simulink model "notch"  (R2017a)
settings: Solver=VariableStepAuto  StartTime=0.0  StopTime=20  RelTol=1e-3
settings Model: Creator=Chaohua Zhao  LastModifiedBy=Chaohua Zhao

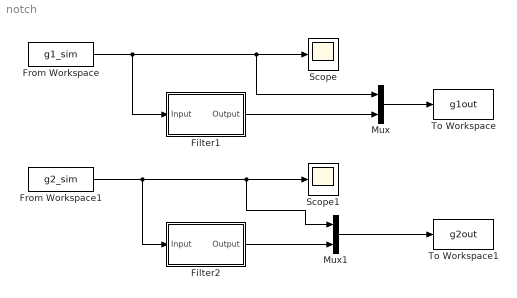
== system notch ==
  Filter1 : Subsystem  Tag=FilterWizardSubSystem
      settings: ErrorFcn=dspFilterRealizedInBasicElemsAlgLoopErrFcnCallback
  Filter2 : Subsystem  Tag=FilterWizardSubSystem
      settings: ErrorFcn=dspFilterRealizedInBasicElemsAlgLoopErrFcnCallback
  From Workspace : FromWorkspace  VariableName=g1_sim  SampleTime=0.001  OutputAfterFinalValue=Setting to zero
  From Workspace1 : FromWorkspace  VariableName=g2_sim  SampleTime=0.001  OutputAfterFinalValue=Setting to zero
  Mux : Mux  Inputs=2
  Mux1 : Mux  Inputs=2
  Scope : Scope
  Scope1 : Scope
  To Workspace : ToWorkspace  VariableName=g1out  SampleTime=-1
  To Workspace1 : ToWorkspace  VariableName=g2out  SampleTime=-1
  wires:
  From Workspace/1 -> Filter1/1(Input), Mux/1, Scope/1
  Filter1/1(Output) -> Mux/2
  Mux/1 -> To Workspace/1
  Filter2/1(Output) -> Mux1/2
  From Workspace1/1 -> Filter2/1(Input), Mux1/1, Scope1/1
  Mux1/1 -> To Workspace1/1

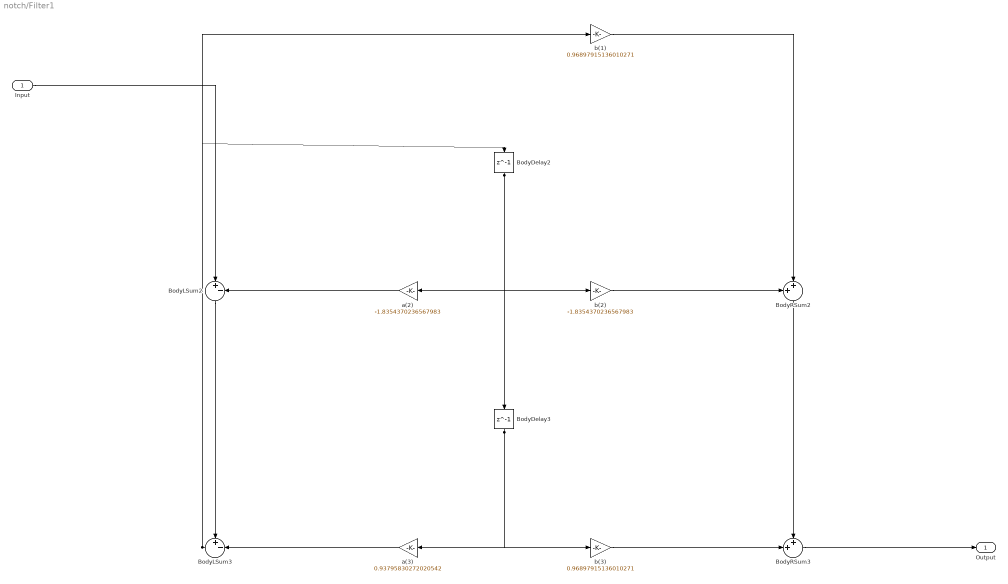
== system notch/Filter1 ==
  Input : Inport
  BodyDelay2 : Delay  DelayLength=1  InitialCondition=0
  BodyDelay3 : Delay  DelayLength=1  InitialCondition=0
  BodyLSum2 : Sum  Inputs=|+-  RndMeth=Nearest  SaturateOnIntegerOverflow=on  OutDataTypeStr=Inherit: Same as first input
  BodyLSum3 : Sum  Inputs=+-|  RndMeth=Nearest  SaturateOnIntegerOverflow=on  OutDataTypeStr=Inherit: Same as first input
  BodyRSum2 : Sum  Inputs=++|  RndMeth=Nearest  SaturateOnIntegerOverflow=on  OutDataTypeStr=Inherit: Same as first input
  BodyRSum3 : Sum  Inputs=++|  RndMeth=Nearest  SaturateOnIntegerOverflow=on  OutDataTypeStr=Inherit: Same as first input
  a(2) : Gain  Gain=-1.8354370236567983  ParamDataTypeStr=double  RndMeth=Nearest  SaturateOnIntegerOverflow=on  OutDataTypeStr=Inherit: Same as input
  a(3) : Gain  Gain=0.93795830272020542  ParamDataTypeStr=double  RndMeth=Nearest  SaturateOnIntegerOverflow=on  OutDataTypeStr=Inherit: Same as input
  b(1) : Gain  Gain=0.96897915136010271  ParamDataTypeStr=double  RndMeth=Nearest  SaturateOnIntegerOverflow=on  OutDataTypeStr=Inherit: Same as input
  b(2) : Gain  Gain=-1.8354370236567983  ParamDataTypeStr=double  RndMeth=Nearest  SaturateOnIntegerOverflow=on  OutDataTypeStr=Inherit: Same as input
  b(3) : Gain  Gain=0.96897915136010271  ParamDataTypeStr=double  RndMeth=Nearest  SaturateOnIntegerOverflow=on  OutDataTypeStr=Inherit: Same as input
  Output : Outport
  wires:
  BodyRSum3/1 -> Output/1
  b(3)/1 -> BodyRSum3/2
  BodyDelay3/1 -> b(3)/1, a(3)/1
  a(3)/1 -> BodyLSum3/2
  BodyLSum3/1 -> BodyDelay2/1, b(1)/1
  BodyRSum2/1 -> BodyRSum3/1
  b(2)/1 -> BodyRSum2/1
  BodyDelay2/1 -> BodyDelay3/1, b(2)/1, a(2)/1
  a(2)/1 -> BodyLSum2/2
  BodyLSum2/1 -> BodyLSum3/1
  Input/1 -> BodyLSum2/1
  b(1)/1 -> BodyRSum2/2

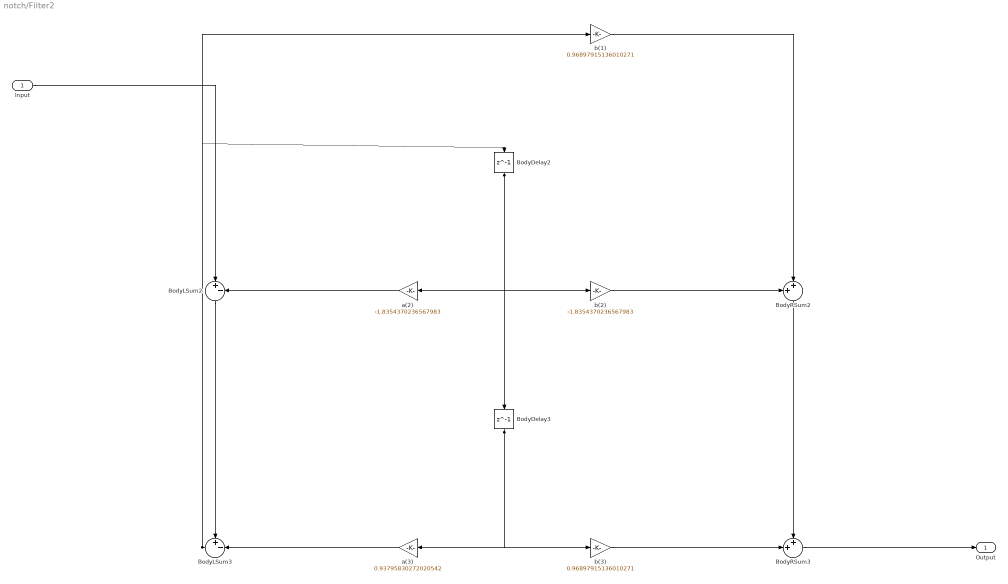
== system notch/Filter2 ==
  Input : Inport
  BodyDelay2 : Delay  DelayLength=1  InitialCondition=0
  BodyDelay3 : Delay  DelayLength=1  InitialCondition=0
  BodyLSum2 : Sum  Inputs=|+-  RndMeth=Nearest  SaturateOnIntegerOverflow=on  OutDataTypeStr=Inherit: Same as first input
  BodyLSum3 : Sum  Inputs=+-|  RndMeth=Nearest  SaturateOnIntegerOverflow=on  OutDataTypeStr=Inherit: Same as first input
  BodyRSum2 : Sum  Inputs=++|  RndMeth=Nearest  SaturateOnIntegerOverflow=on  OutDataTypeStr=Inherit: Same as first input
  BodyRSum3 : Sum  Inputs=++|  RndMeth=Nearest  SaturateOnIntegerOverflow=on  OutDataTypeStr=Inherit: Same as first input
  a(2) : Gain  Gain=-1.8354370236567983  ParamDataTypeStr=double  RndMeth=Nearest  SaturateOnIntegerOverflow=on  OutDataTypeStr=Inherit: Same as input
  a(3) : Gain  Gain=0.93795830272020542  ParamDataTypeStr=double  RndMeth=Nearest  SaturateOnIntegerOverflow=on  OutDataTypeStr=Inherit: Same as input
  b(1) : Gain  Gain=0.96897915136010271  ParamDataTypeStr=double  RndMeth=Nearest  SaturateOnIntegerOverflow=on  OutDataTypeStr=Inherit: Same as input
  b(2) : Gain  Gain=-1.8354370236567983  ParamDataTypeStr=double  RndMeth=Nearest  SaturateOnIntegerOverflow=on  OutDataTypeStr=Inherit: Same as input
  b(3) : Gain  Gain=0.96897915136010271  ParamDataTypeStr=double  RndMeth=Nearest  SaturateOnIntegerOverflow=on  OutDataTypeStr=Inherit: Same as input
  Output : Outport
  wires:
  b(1)/1 -> BodyRSum2/2
  Input/1 -> BodyLSum2/1
  BodyLSum2/1 -> BodyLSum3/1
  a(2)/1 -> BodyLSum2/2
  BodyDelay2/1 -> a(2)/1, b(2)/1, BodyDelay3/1
  b(2)/1 -> BodyRSum2/1
  BodyRSum2/1 -> BodyRSum3/1
  BodyLSum3/1 -> b(1)/1, BodyDelay2/1
  a(3)/1 -> BodyLSum3/2
  BodyDelay3/1 -> a(3)/1, b(3)/1
  b(3)/1 -> BodyRSum3/2
  BodyRSum3/1 -> Output/1
